simulink model "potenlab"  (R2024b)
settings: Solver=FixedStepAuto  StartTime=0.0  StopTime=10  FixedStep=1  RelTol=1e-3  EnableMultiTasking=on
libraries: stm32f4xxblockslib x2, dspstat3 x2, spsCurrentMeasurementLib x1, spsDCVoltageSourceLib x1, simulink x1, spsGroundLib x1, spsIdealSwitchLib x1, spsSeriesRLCBranchLib x1, spspowerguiLib x1
(part 2 of 2)

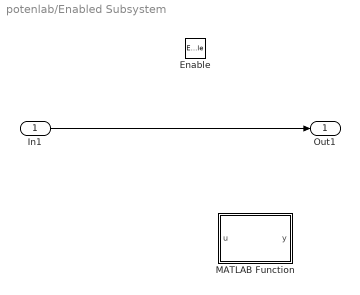
== system potenlab/Enabled Subsystem ==
  In1 : Inport
  Enable : EnablePort
  MATLAB Function : MATLAB Function  TreatAsAtomicUnit=on
  Out1 : Outport
  wires:
  In1/1 -> Out1/1

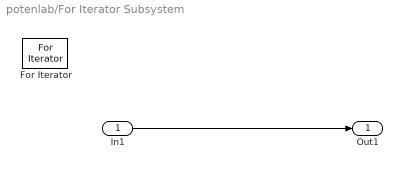
== system potenlab/For Iterator Subsystem ==
  In1 : Inport
  For Iterator : ForIterator
  Out1 : Outport
  wires:
  In1/1 -> Out1/1

== matlab function potenlab/Enabled Subsystem/MATLAB Function ==
  data: u input; y output
function y = fcn(u)

for i = 1:length(10):
y = u;
